simulink model "PID"  (R2017b)
settings: Solver=VariableStepAuto  StartTime=0.0  StopTime=1  RelTol=1e-3
settings Model: Creator=黄洋  LastModifiedBy=黄洋

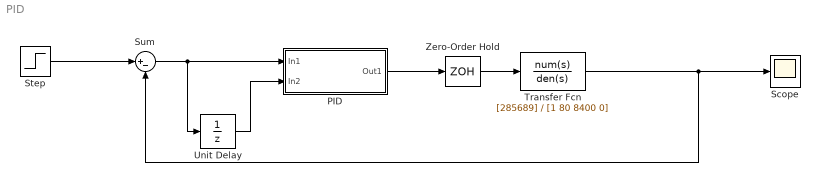
== system PID ==
  PID : Subsystem
  Scope : Scope
  Step : Step  Time=0  SampleTime=0
  Sum : Sum  Inputs=|+-
  Transfer Fcn : TransferFcn  Numerator=[285689]  Denominator=[1 80 8400 0]
  Unit Delay : UnitDelay  SampleTime=0.001
  Zero-Order Hold : ZeroOrderHold  SampleTime=-1
  wires:
  Step/1 -> Sum/1
  Sum/1 -> Unit Delay/1, PID/1(In1)
  Transfer Fcn/1 -> Sum/2, Scope/1
  Unit Delay/1 -> PID/2(In2)
  PID/1(Out1) -> Zero-Order Hold/1
  Zero-Order Hold/1 -> Transfer Fcn/1

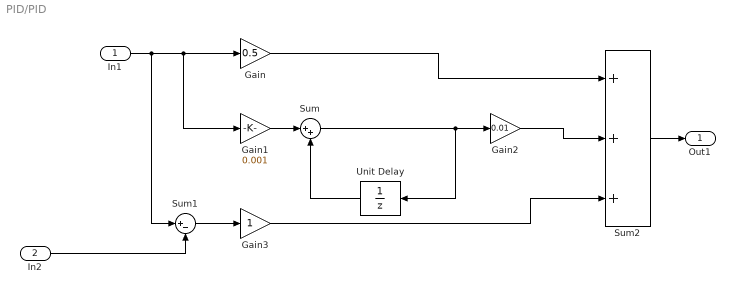
== system PID/PID ==
  In1 : Inport
  In2 : Inport  Port=2
  Gain : Gain  Gain=0.5
  Gain1 : Gain  Gain=0.001
  Gain2 : Gain  Gain=0.01
  Gain3 : Gain
  Sum : Sum  Inputs=|++
  Sum1 : Sum  Inputs=|+-
  Sum2 : Sum  Inputs=+++
  Unit Delay : UnitDelay  SampleTime=0.001
  Out1 : Outport
  wires:
  In1/1 -> Sum1/1, Gain1/1, Gain/1
  Gain1/1 -> Sum/1
  Sum/1 -> Gain2/1, Unit Delay/1
  Unit Delay/1 -> Sum/2
  Gain/1 -> Sum2/1
  Gain2/1 -> Sum2/2
  In2/1 -> Sum1/2
  Sum1/1 -> Gain3/1
  Gain3/1 -> Sum2/3
  Sum2/1 -> Out1/1
